simulink model "ExampleC1"  (Simulink 8.6)
settings: Solver=ode45  StartTime=0.0  StopTime=3  RelTol=1e-3
settings Model: Creator=Jacques-Ezechiel  LastModifiedBy=Jacques-Ezechiel
settings DataIOCC: SaveFormat=Dataset  SignalLoggingSaveFormat=Dataset
settings OptimizationCC: ExpressionDepthLimit=128
settings DebuggingCC: UnderspecifiedInitializationDetection=Simplified  MergeDetectMultiDrivingBlocksExec=error  SolverPrmCheckMsg=none  FcnCallInpInsideContextMsg=EnableAllAsError  StateNameClashWarn=none
settings HardwareCC: ProdBitPerPointer=64  ProdLargestAtomicFloat=Float  ProdIntDivRoundTo=Zero  ProdEndianess=LittleEndian  ProdWordSize=64  ProdHWDeviceType=Intel->x86-64 (Windows64)
settings GRTTargetCC: GeneratePreprocessorConditionals=Use local settings  CombineOutputUpdateFcns=on  GRTInterface=off
settings ConfigComp: CovModelRefEnable=off

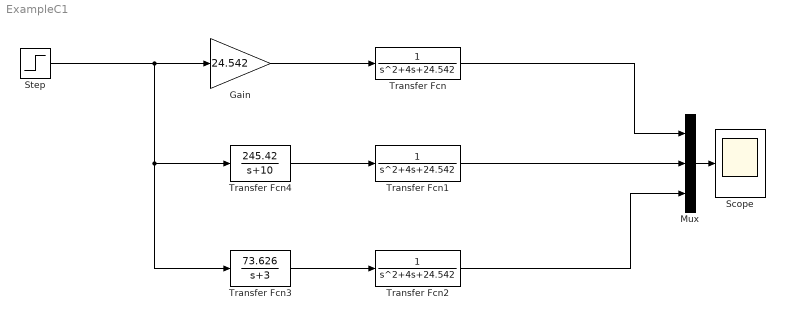
== system ExampleC1 ==
  Gain : Gain  Gain=24.542
  Mux : Mux  Inputs=3
  Scope : Scope
  Step : Step  Time=0  SampleTime=0
  Transfer Fcn : TransferFcn  Denominator=[1 4 24.542]
  Transfer Fcn1 : TransferFcn  Denominator=[1 4 24.542]
  Transfer Fcn2 : TransferFcn  Denominator=[1 4 24.542]
  Transfer Fcn3 : TransferFcn  Numerator=[73.626]  Denominator=[1 3]
  Transfer Fcn4 : TransferFcn  Numerator=[245.42]  Denominator=[1 10]
  wires:
  Mux/1 -> Scope/1
  Gain/1 -> Transfer Fcn/1
  Transfer Fcn4/1 -> Transfer Fcn1/1
  Transfer Fcn3/1 -> Transfer Fcn2/1
  Transfer Fcn2/1 -> Mux/3
  Transfer Fcn1/1 -> Mux/2
  Transfer Fcn/1 -> Mux/1
  Step/1 -> Transfer Fcn3/1, Transfer Fcn4/1, Gain/1
